simulink model "mCloneDetectionAPI3"  (R2022a)
settings: Solver=FixedStepDiscrete  StartTime=0.0  StopTime=10.0  FixedStep=1  RelTol=1e-3  EnableMultiTasking=on
PreLoadFcn:
  | A=Simulink.Parameter;
  | A.Value=9;
  | B=Simulink.Parameter;
  | B.Value=9;
  | 
  | V = Simulink.Parameter;
  | V.CoderInfo.StorageClass = 'custom';
  | V.CoderInfo.CustomStorageClass = 'CompilerFlag';
  | V.Value = 1;
  | V.DataType = 'int32';
  | 
  | W = Simulink.Parameter;
  | W.CoderInfo.StorageClass = 'custom';
  | W.CoderInfo.CustomStorageClass = 'CompilerFlag';
  | W.Value = 2;
  | W.DataType = 'int32';
model workspace (MAT data in the model file):
  C = Simulink.Parameter
  C.DataType = 'auto'
  C.Complexity = 'real'
  C.Dimensions = [0 0]
Description:
  | Use this model in conjunction with the library ex_clone_library to show how the Identify Modeling Clones tool works.
  | For more information, see the example Enable Component Reuse with Clone Detection.
settings Model: Creator=The MathWorks, Inc.  LastModifiedBy=ssinghal
settings SolverCC: AlgebraicLoopSolver=TrustRegion  MaxZcPerStep=1
settings DataIOCC: LimitDataPoints=on  SaveFormat=Array  SaveOutput=off  SaveTime=off  ReturnWorkspaceOutputs=off
settings OptimizationCC: DefaultParameterBehavior=Inlined  UseDivisionForNetSlopeComputation=on  InlineInvariantSignals=on  EnhancedBackFolding=on  StateBitsets=on  DataBitsets=on  EfficientFloat2IntCast=on
settings DebuggingCC: UnderspecifiedInitializationDetection=Classic  MergeDetectMultiDrivingBlocksExec=none  UnconnectedInputMsg=warning  UnconnectedOutputMsg=warning  UnconnectedLineMsg=warning  AllowSymbolicDim=off  SFUnexpectedBacktrackingDiag=warning  SFNoUnconditionalDefaultTransitionDiag=warning  SFExecutionAtInitializationDiag=none  SFMachineParentedDataDiag=warning  ArithmeticOperatorsInVariantConditions=warning
settings HardwareCC: TargetIntDivRoundTo=Zero  TargetEndianess=LittleEndian  TargetHWDeviceType=Generic->32-bit Embedded Processor
settings ModelReferenceCC: PropagateSignalLabelsOutOfModel=off
settings SFSimCC: SimUseLocalCustomCode=off  CustomCodeUndefinedFunction=UseInterfaceOnly
settings RTWCC: Description=Generic Real-Time Target  GenerateReport=on  RTWVerbose=off  RTWUseLocalCustomCode=off  LaunchReport=on  DLArmComputeVersion=19.05
settings CodeAppCC: ForceParamTrailComments=on  StateflowObjectComments=on
settings GRTTargetCC: TargetLangStandard=C89/C90 (ANSI)
settings ConfigComp: CovMetricSettings=dw  CovSaveCumulativeToWorkspaceVar=on  CovSaveSingleToWorkspaceVar=on  CovExternalEMLEnable=off  CovSFcnEnable=off

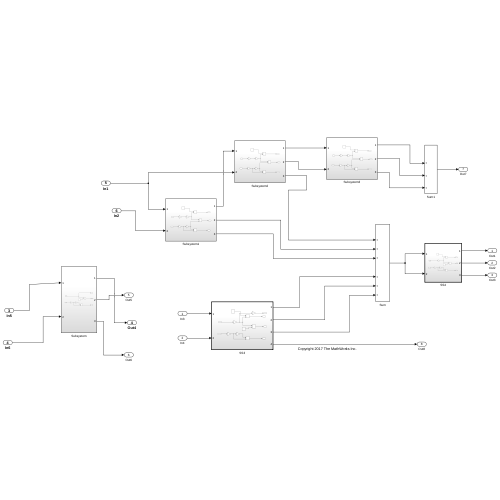
[thumbnail: Simulink's stored preview of the top-level diagram]
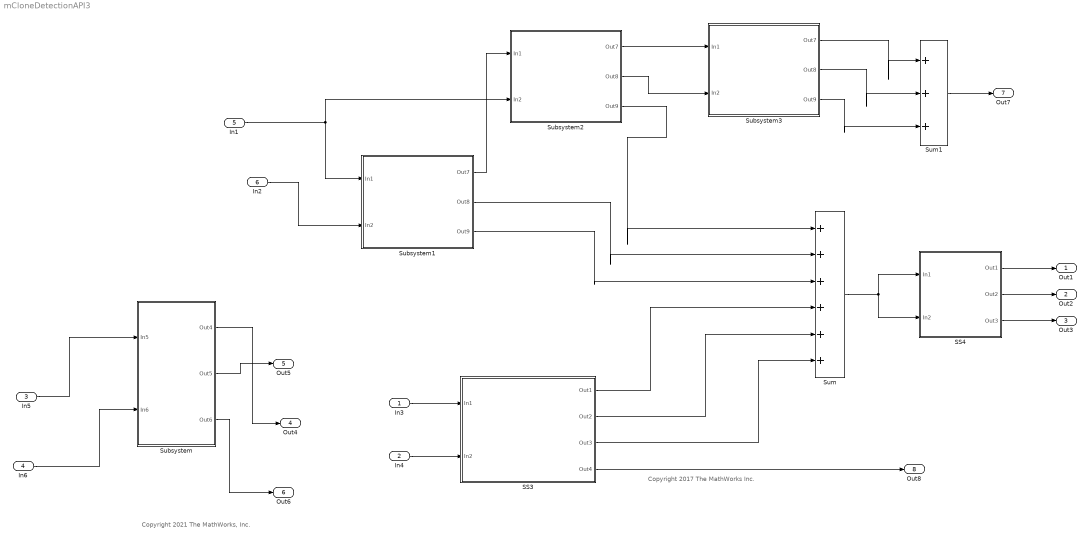
== system mCloneDetectionAPI3 ==
  note: Copyright 2017 The MathWorks Inc.
  note: Copyright 2021 The MathWorks, Inc.
  In3 : Inport
  In4 : Inport  Port=2
  In5 : Inport  Port=3
  In6 : Inport  Port=4
  In1 : Inport  Port=5
  In2 : Inport  Port=6
  SS3 : Subsystem  TreatAsAtomicUnit=on
  SS4 : Subsystem  TreatAsAtomicUnit=on
  Subsystem : Subsystem
  Subsystem1 : Subsystem
  Subsystem2 : Subsystem
  Subsystem3 : Subsystem
  Sum : Sum  Inputs=|+++|+++
  Sum1 : Sum  Inputs=|+++
  Out1 : Outport
  Out2 : Outport  Port=2
  Out3 : Outport  Port=3
  Out4 : Outport  Port=4  VectorParamsAs1DForOutWhenUnconnected=off
  Out5 : Outport  Port=5
  Out6 : Outport  Port=6
  Out7 : Outport  Port=7
  Out8 : Outport  Port=8
  wires:
  Subsystem2/3(Out9) -> Sum/1
  In3/1 -> SS3/1(In1)
  In5/1 -> Subsystem/1(In5)
  Subsystem/3(Out6) -> Out6/1
  SS4/3(Out3) -> Out3/1
  In6/1 -> Subsystem/2(In6)
  Subsystem/2(Out5) -> Out5/1
  Subsystem/1(Out4) -> Out4/1
  SS4/1(Out1) -> Out1/1
  SS3/3(Out3) -> Sum/6
  SS3/2(Out2) -> Sum/5
  Subsystem1/3(Out9) -> Sum/3
  Subsystem1/2(Out8) -> Sum/2
  Sum/1 -> SS4/1(In1), SS4/2(In2)
  In4/1 -> SS3/2(In2)
  SS3/1(Out1) -> Sum/4
  SS4/2(Out2) -> Out2/1
  In1/1 -> Subsystem2/2(In2), Subsystem1/1(In1)
  In2/1 -> Subsystem1/2(In2)
  Subsystem1/1(Out7) -> Subsystem2/1(In1)
  Subsystem2/2(Out8) -> Subsystem3/2(In2)
  Subsystem2/1(Out7) -> Subsystem3/1(In1)
  Subsystem3/1(Out7) -> Sum1/1
  Subsystem3/2(Out8) -> Sum1/2
  Subsystem3/3(Out9) -> Sum1/3
  Sum1/1 -> Out7/1
  SS3/4(Out4) -> Out8/1

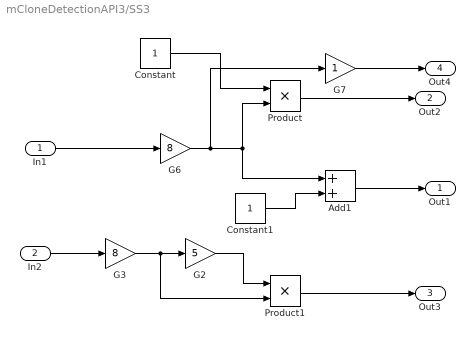
== system mCloneDetectionAPI3/SS3 ==
  In1 : Inport
  In2 : Inport  Port=2
  Add1 : Sum
  Constant : Constant
  Constant1 : Constant
  G2 : Gain  Gain=5
  G3 : Gain  Gain=8
  G6 : Gain  Gain=8
  G7 : Gain
  Product : Product
  Product1 : Product
  Out1 : Outport  VectorParamsAs1DForOutWhenUnconnected=off
  Out2 : Outport  Port=2
  Out3 : Outport  Port=3
  Out4 : Outport  Port=4
  wires:
  Constant/1 -> Product/1
  Add1/1 -> Out1/1
  G6/1 -> G7/1, Add1/1, Product/2
  Product/1 -> Out2/1
  G3/1 -> Product1/2, G2/1
  In1/1 -> G6/1
  Product1/1 -> Out3/1
  In2/1 -> G3/1
  Constant1/1 -> Add1/2
  G2/1 -> Product1/1
  G7/1 -> Out4/1

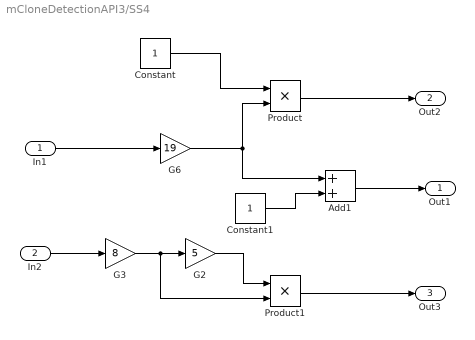
== system mCloneDetectionAPI3/SS4 ==
  In1 : Inport
  In2 : Inport  Port=2
  Add1 : Sum
  Constant : Constant
  Constant1 : Constant
  G2 : Gain  Gain=5
  G3 : Gain  Gain=8
  G6 : Gain  Gain=19
  Product : Product
  Product1 : Product
  Out1 : Outport  VectorParamsAs1DForOutWhenUnconnected=off
  Out2 : Outport  Port=2
  Out3 : Outport  Port=3
  wires:
  G2/1 -> Product1/1
  Constant1/1 -> Add1/2
  In2/1 -> G3/1
  Product1/1 -> Out3/1
  In1/1 -> G6/1
  G3/1 -> G2/1, Product1/2
  Product/1 -> Out2/1
  G6/1 -> Product/2, Add1/1
  Add1/1 -> Out1/1
  Constant/1 -> Product/1

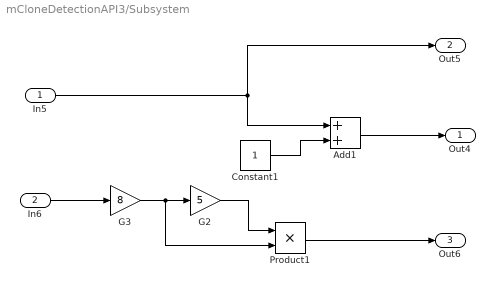
== system mCloneDetectionAPI3/Subsystem ==
  In5 : Inport
  In6 : Inport  Port=2
  Add1 : Sum
  Constant1 : Constant
  G2 : Gain  Gain=5
  G3 : Gain  Gain=8
  Product1 : Product
  Out4 : Outport  VectorParamsAs1DForOutWhenUnconnected=off
  Out5 : Outport  Port=2
  Out6 : Outport  Port=3
  wires:
  G3/1 -> G2/1, Product1/2
  G2/1 -> Product1/1
  In5/1 -> Out5/1, Add1/1
  Product1/1 -> Out6/1
  Constant1/1 -> Add1/2
  In6/1 -> G3/1
  Add1/1 -> Out4/1

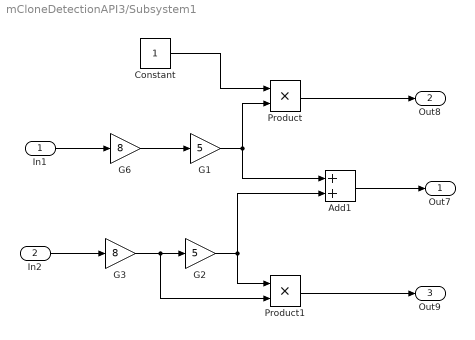
== system mCloneDetectionAPI3/Subsystem1 ==
  In1 : Inport
  In2 : Inport  Port=2
  Add1 : Sum
  Constant : Constant
  G1 : Gain  Gain=5
  G2 : Gain  Gain=5
  G3 : Gain  Gain=8
  G6 : Gain  Gain=8
  Product : Product
  Product1 : Product
  Out7 : Outport  VectorParamsAs1DForOutWhenUnconnected=off
  Out8 : Outport  Port=2
  Out9 : Outport  Port=3
  wires:
  Add1/1 -> Out7/1
  Constant/1 -> Product/1
  Product1/1 -> Out9/1
  G1/1 -> Add1/1, Product/2
  G3/1 -> Product1/2, G2/1
  G2/1 -> Product1/1, Add1/2
  Product/1 -> Out8/1
  In1/1 -> G6/1
  G6/1 -> G1/1
  In2/1 -> G3/1

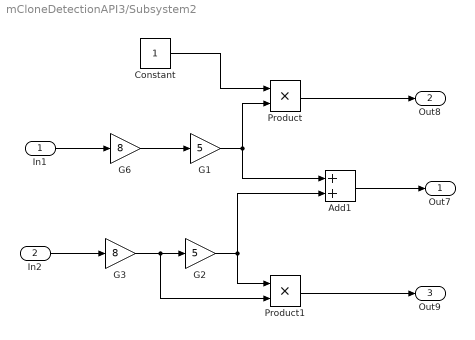
== system mCloneDetectionAPI3/Subsystem2 ==
  In1 : Inport
  In2 : Inport  Port=2
  Add1 : Sum
  Constant : Constant
  G1 : Gain  Gain=5
  G2 : Gain  Gain=5
  G3 : Gain  Gain=8
  G6 : Gain  Gain=8
  Product : Product
  Product1 : Product
  Out7 : Outport  VectorParamsAs1DForOutWhenUnconnected=off
  Out8 : Outport  Port=2
  Out9 : Outport  Port=3
  wires:
  In2/1 -> G3/1
  G6/1 -> G1/1
  In1/1 -> G6/1
  Product/1 -> Out8/1
  G2/1 -> Add1/2, Product1/1
  G3/1 -> G2/1, Product1/2
  G1/1 -> Product/2, Add1/1
  Product1/1 -> Out9/1
  Constant/1 -> Product/1
  Add1/1 -> Out7/1

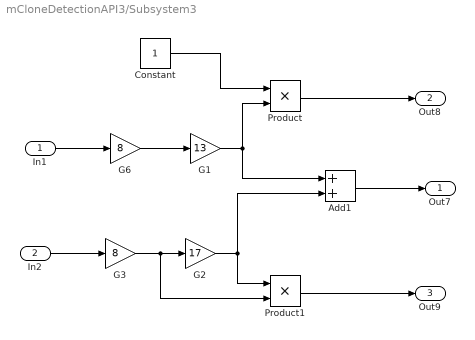
== system mCloneDetectionAPI3/Subsystem3 ==
  In1 : Inport
  In2 : Inport  Port=2
  Add1 : Sum
  Constant : Constant
  G1 : Gain  Gain=13
  G2 : Gain  Gain=17
  G3 : Gain  Gain=8
  G6 : Gain  Gain=8
  Product : Product
  Product1 : Product
  Out7 : Outport  VectorParamsAs1DForOutWhenUnconnected=off
  Out8 : Outport  Port=2
  Out9 : Outport  Port=3
  wires:
  In2/1 -> G3/1
  G6/1 -> G1/1
  In1/1 -> G6/1
  Product/1 -> Out8/1
  G2/1 -> Add1/2, Product1/1
  G3/1 -> G2/1, Product1/2
  G1/1 -> Product/2, Add1/1
  Product1/1 -> Out9/1
  Constant/1 -> Product/1
  Add1/1 -> Out7/1
